simulink model "pg"  (R2021a)
settings: Solver=VariableStepAuto  StartTime=0.0  StopTime=10.0  RelTol=1e-3
settings Model: Creator=61301765  LastModifiedBy=61301765

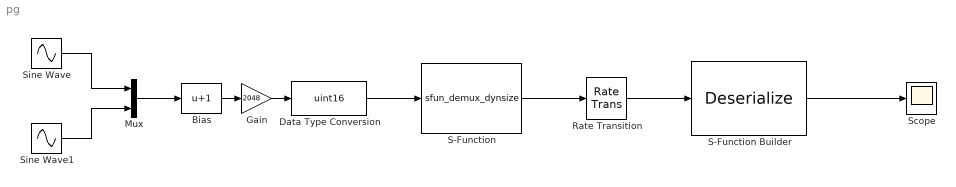
== system pg ==
  Bias : Bias  Bias=1
  Data Type Conversion : DataTypeConversion  OutDataTypeStr=uint16
  Gain : Gain  Gain=2048
  Mux : Mux  Inputs=2
  Rate Transition : RateTransition  OutPortSampleTime=1/40e3
  S-Function : S-Function  FunctionName=sfun_demux_dynsize  SFunctionDeploymentMode=off  EnableBusSupport=off
  S-Function Builder : S-Function  FunctionName=Deserialize  SFunctionModules=Deserialize_wrapper  SFunctionDeploymentMode=off  EnableBusSupport=off  mask(S-Function Builder){}
      mask help: Simulink:masks:SFunctionBuilder_MD
      mask init:
      | val = [[.9  0.75 0.75 1 1 .9 .9 1]',[1 1 0.75 0.75 .9 .9 1 .9]'];try , sys = get_param(gcb,'SfunBuilderFcnName');if isempty(sys), sys = get_param(gcb,'FunctionName'); end,catch, sys = get_param(gcb,'FunctionName'); end
      settings: CopyFcn=set_param(gcbh,'LinkStatus','none')  OpenFcn=sfunctionwizard(gcbh)
      mask Display: plot(val(:,1),val(:,2)),disp(sys),port_label('input',1,'u0'),port_label('output',1,'y0')
  Scope : Scope
  Sine Wave : Sin  Phase=pi/2  SampleTime=1/20e3
  Sine Wave1 : Sin  SampleTime=1/20e3
  wires:
  Bias/1 -> Gain/1
  Gain/1 -> Data Type Conversion/1
  Sine Wave/1 -> Mux/1
  Sine Wave1/1 -> Mux/2
  Mux/1 -> Bias/1
  S-Function Builder/1 -> Scope/1
  Data Type Conversion/1 -> S-Function/1
  S-Function/1 -> Rate Transition/1
  Rate Transition/1 -> S-Function Builder/1
